simulink model "stateflow_internaltransition"  (R2016b)
settings: Solver=VariableStepAuto  StartTime=0.0  StopTime=10.0  RelTol=1e-3  EnableMultiTasking=on
settings Model: Creator=amyyang  LastModifiedBy=amyyang
settings DataIOCC: LimitDataPoints=on
settings OptimizationCC: LifeSpan=inf
settings DebuggingCC: AllowSymbolicDim=off  SFUnexpectedBacktrackingDiag=warning  SFNoUnconditionalDefaultTransitionDiag=warning  SFExecutionAtInitializationDiag=none
settings ModelReferenceCC: PropagateSignalLabelsOutOfModel=off
settings GRTTargetCC: TargetLangStandard=C89/C90 (ANSI)
settings ConfigComp: CovMetricSettings=dw  CovHtmlReporting=on  CovSaveCumulativeToWorkspaceVar=on  CovSaveSingleToWorkspaceVar=on  CovExternalEMLEnable=off

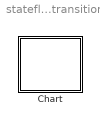
== system stateflow_internaltransition ==
  Chart : Stateflow chart  TreatAsAtomicUnit=on

== stateflow chart stateflow_internaltransition/Chart ==
  state a1
    entry:
    t1 = 0;
    entry,during:
    t1++;
    during:
    t1++;
  state a
    entry:
    t1 = 0;
    during:
    t1++;
    (default) -> (junction 111)
    a -> (junction 111)
    (junction 111) -> (junction 114) : { t1++;}
  note: 6.2 强烈建立 在 State 内部
      | 不要混用 流程图 和 en、du,ex等语句。
      | 因为这样执行顺序不直观。
  state a2
    (default) -> (junction 128) : {
        |  t2 = 0;
        | }
    a2 -> (junction 128) [order 1] : {
        | t2++;
        | }
    (junction 128) -> (junction 125) : {
        | t2++;
        | }
  state a3
    entry:
    t2 = 0;
    during:
    t2++;
    (default) -> (junction 138)
    a3 -> (junction 138) [order 1]
    (junction 138) -> (junction 136) : {
        | t2++;
        | }
  note: 6.1 强烈建议 所有的状态的内部跳转连线
      | 必须在 State 框线的左侧面。
  state State1
    state A
    state B
    state C
    (default) -> A
    State1 -> (junction 81)
    (junction 81) -> A [order 1] : [C1]
    (junction 81) -> (junction 84) [order 2]
    (junction 84) -> B [order 1] : [C2]
    (junction 84) -> (junction 85) [order 2]
    (junction 85) -> C : [C3]
  state State2
    state AA
    state AB
    state AC
    (default) -> AA
    State2 -> AA [order 1] : [C1]
    State2 -> AB [order 2] : [C2]
    State2 -> AC [order 3] : [C3]
  note: 6.3~4 建议同一个 state 最好不要有多个内部跳转。
      | 如果有多个内部跳转，
      | 强烈建议 跳转线按照从上到下的优先级设置。
  state State3
    state ?
    state ?
    state ?
    (default) -> State3.?
    State3 -> State3.? [order 1] : [C1]
    State3 -> State3.? [order 2] : [C2]
    State3 -> State3.? [order 3] : [C3]
  state Incorrect
    state ?
    state ?
    state ?
    (default) -> Incorrect.?
    Incorrect -> Incorrect.? [order 1] : [C1]
    Incorrect -> Incorrect.? [order 3] : [C2]
    Incorrect -> Incorrect.? [order 2] : [C3]
  note: 如果一定要有多个跳转，
      | 则一定要从上到下的排列
  (default) -> a1 [order 1]
  (default) -> a [order 2]
  a1 -> a2 : [ t1 >= 100]
  a2 -> a1 [order 1] : [ t2 >= 100]
  (default) -> a3 [order 3] : [ t1 >= 100]
  a3 -> a [order 1] : [ t2 >= 100]
  (default) -> State1 [order 4]
  (default) -> State2 [order 5]
